simulink model "Hexa_ASMC"  (R2023a)
settings: Solver=ode4  StartTime=0.0  StopTime=tf  FixedStep=0.01  RelTol=1e-3
values from neighbouring files (symbols this model uses):
  ArmConstants = struct('l1_dim', l1_dim,                        'l2_dim', l2_dim,                        'Hexa_to_joint_L', L,                        'Mass1', ml1,                        'Mass2', ml2,                        'Inertia1', Hl1,                        'Inertia2', Hl2,                        'MC1', c1,                        'MC2', c2,                        'Servos', Servos)    [init_model.m]
  HexaConstants = struct('Mass', mb,                         'Inertia', J ,                         'invallo', invallo,                         'kT', kT)    [init_model.m]
settings Model: Creator=Jorge  LastModifiedBy=danie
settings DataIOCC: ReturnWorkspaceOutputs=off
settings OptimizationCC: ReuseModelBlockBuffer=off
settings DebuggingCC: UnconnectedInputMsg=warning  UnconnectedOutputMsg=warning  UnconnectedLineMsg=warning
settings ModelReferenceCC: EnableRefExpFcnMdlSchedulingChecks=on
settings RTWCC: DLArmComputeVersion=19.05
settings DiagnosticsConfigSet: SimMechanicsRigidlyBoundBlock=warning
settings ExplorerConfigSet: InternalSimMechanicsExplorerSettings="<ExplorerConfiguration><canonicalview>default</canonicalview><AnimationSetting><BasePlaybackSpeed>1.0</BasePlaybackSpeed><PlaybackSpeedFactor>4.0</PlaybackSpeedFactor></AnimationSetting><TilePanel><TileInfo><Tiles Columns=\"1\" Count=\"1\" Rows=\"1\"><Column Weight=\"1\"/><Row Weight=\"1\"/><Tile Height=\"1\" Width=\"1\" X=\"0\" Y=\"0\"/></Tiles></TileInfo><SceneInfo><SceneViewer><BGColor><R>0.60000002384185791</R><G>0.60000002384185791</G><B>0.60000002384185791</B></BGColor><Camera><DoPerspective>off</DoPerspective><Position><X>-3.90727997960079421</X><Y>2.05428323506579513</Y><Z>1.78515478561793706</Z></Position><Center><X>0.0641025917185230748</X><Y>-0.340203768406677431</Y><Z>0.439985738763349676</Z></Center><Up><X>0.2129099347365212</X><Y>-0.185763056293179685</Y><Z>0.959250460832366536</Z></Up><ViewLimDist>1</ViewLimDist><YLim>1.44101175579229102</YLim><XLim>2.86953370221693493</XLim></Camera></SceneViewer></SceneInfo></TilePanel><MechEditorPanel><Cameras/><GfxPanelCameraMap/><VideoCreator><PlaybackSpeedRatio>4.0</PlaybackSpeedRatio><FrameRate>30</FrameRate><VideoFormat>MPEG-4</VideoFormat><FrameSize>[1920 1080]</FrameSize></VideoCreator></MechEditorPanel></ExplorerConfiguration>"

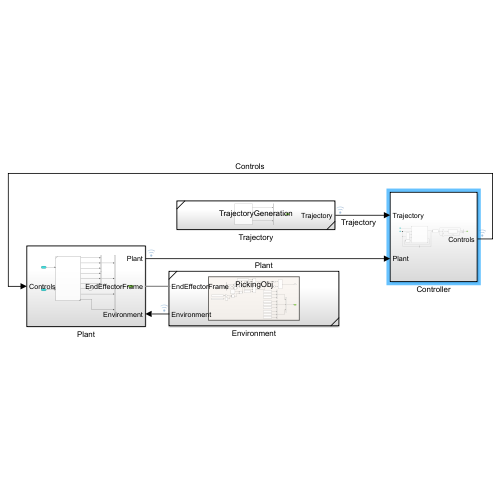
[thumbnail: Simulink's stored preview of the top-level diagram]
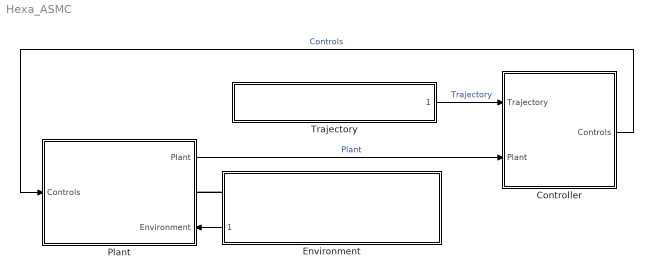
== system Hexa_ASMC ==
  Controller : Subsystem
  Environment : Subsystem  ReferencedSubsystem=PickingObj
      settings: PortSchema="{\"entries\":[{\"content\":{\"sides\":[{\"content\":{\"connectorIds\":[\"LConn1\",\"Out1\"]},\"type\":\"ConnectorPlacement.EquallySpacedRectSide\",\"uuid\":\"5c08cfce-bb37-47ad-9aee-09cd3d0a9d82\"},{\"content\":{\"side\":\"RIGHT\"},\"type\":\"ConnectorPlacement.EquallySpacedRectSide\",\"uuid\":\"54293c39-26a9-438b-b1f6-8d0b93a0680a\"},{\"content\":{\"side\":\"TOP\"},\"type\":\"ConnectorPlacement.EquallySpacedRectSide\",\"uuid\":\"14552c0b-480b-4ef8-a964-bf21c28e2914\"}]},\"type\":\"ConnectorPlacement.EquallySpacedConnector\",\"uuid\":\"e6e3027e-622b-4c2e-b3cf-73a625fb57e1\"}],\"packageUris\":[\"http://schema.mathworks.com/mf0/Connector/R2020b\"],\"version\":\"1.0\"}"
  Plant : Subsystem
      settings: PortSchema="{\"entries\":[{\"content\":{\"sides\":[{\"content\":{\"connectorIds\":[\"In1\"]},\"type\":\"ConnectorPlacement.EquallySpacedRectSide\",\"uuid\":\"11bcd53b-55b2-4d69-a1dd-85bd17ae1b26\"},{\"content\":{\"connectorIds\":[\"Out1\",\"RConn1\",\"In2\"],\"side\":\"RIGHT\"},\"type\":\"ConnectorPlacement.EquallySpacedRectSide\",\"uuid\":\"8deb2c99-cdf2-4c07-9bda-82202a10127f\"},{\"content\":{\"side\":\"TOP\"},\"type\":\"ConnectorPlacement.EquallySpacedRectSide\",\"uuid\":\"e1cee1e1-f12a-4bbb-be1b-b1297a2f8e40\"}]},\"type\":\"ConnectorPlacement.EquallySpacedConnector\",\"uuid\":\"11daab03-d64c-4920-b3ce-5e6ee12e0c1c\"}],\"packageUris\":[\"http://schema.mathworks.com/mf0/Connector/R2020b\"],\"version\":\"1.0\"}"
  Trajectory : Subsystem  ReferencedSubsystem=TrajectoryGeneration
  wires:
  Trajectory/1 -> Controller/1(Trajectory)  "Trajectory"
  Controller/1(Controls) -> Plant/1(Controls)  "Controls"
  Plant/1(Plant) -> Controller/2(Plant)  "Plant"
  Environment/1 -> Plant/2(Environment)
  connections:
  Environment/LConn1 -- Plant/RConn1

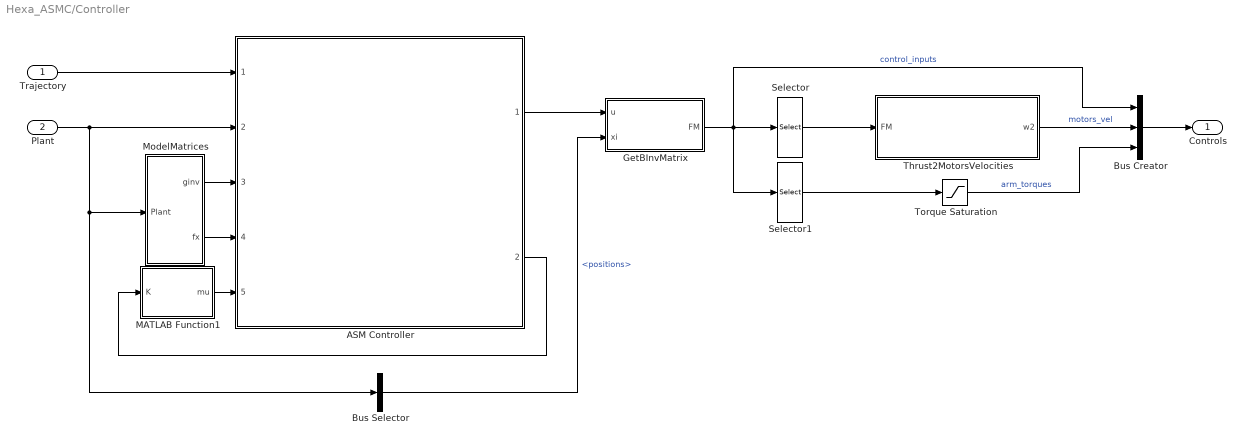
== system Hexa_ASMC/Controller ==
  Trajectory : Inport
  Plant : Inport  Port=2  OutDataTypeStr=Bus: PlantBusDef
  ASM Controller : Subsystem  ReferencedSubsystem=ASMController
  Bus Creator : BusCreator  Inputs=3
  Bus Selector : BusSelector  OutputSignals=positions
  GetBInvMatrix : MATLAB Function  TreatAsAtomicUnit=on
  MATLAB Function1 : MATLAB Function  TreatAsAtomicUnit=on
  ModelMatrices : Subsystem
  Selector : Selector  InputPortWidth=8  IndexOptions=Index vector (dialog)  Indices=1:6  OutputSizes=1
  Selector1 : Selector  InputPortWidth=8  IndexOptions=Index vector (dialog)  Indices=7:8  OutputSizes=1
  Thrust2MotorsVelocities : Subsystem
  Torque Saturation : Saturate  UpperLimit=ArmConstants.Servos.T1max  LowerLimit=-ArmConstants.Servos.T1max
  Controls : Outport  OutDataTypeStr=Bus: ControlsBusDef
  wires:
  Selector/1 -> Thrust2MotorsVelocities/1(FM)
  Selector1/1 -> Torque Saturation/1
  GetBInvMatrix/1(FM) -> Bus Creator/1, Selector1/1, Selector/1  "control_inputs"
  Plant/1 -> Bus Selector/1, ModelMatrices/1(Plant), ASM Controller/2
  Bus Selector/1 -> GetBInvMatrix/2(xi)  "<positions>"
  Torque Saturation/1 -> Bus Creator/3  "arm_torques"
  Thrust2MotorsVelocities/1(w2) -> Bus Creator/2  "motors_vel"
  Bus Creator/1 -> Controls/1
  ASM Controller/2 -> MATLAB Function1/1(K)
  Trajectory/1 -> ASM Controller/1
  ASM Controller/1 -> GetBInvMatrix/1(u)
  ModelMatrices/1(ginv) -> ASM Controller/3
  ModelMatrices/2(fx) -> ASM Controller/4
  MATLAB Function1/1(mu) -> ASM Controller/5

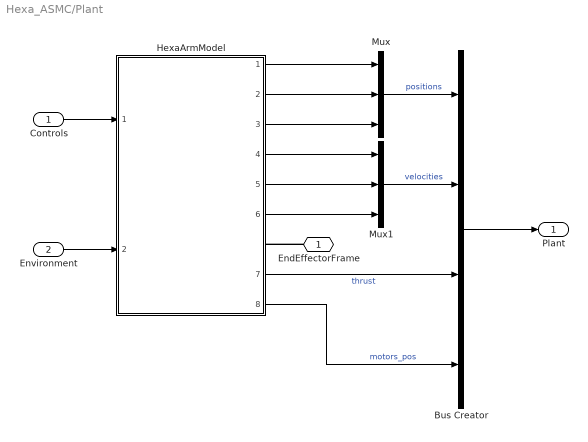
== system Hexa_ASMC/Plant ==
  Controls : Inport  OutDataTypeStr=Bus: ControlsBusDef
  Environment : Inport  Port=2  OutDataTypeStr=Bus: EnvironmentBusDef
  Bus Creator : BusCreator  Inputs=4
  HexaArmModel : Subsystem  ReferencedSubsystem=HexaArmModel
      settings: PortSchema="{\"entries\":[{\"content\":{\"sides\":[{\"content\":{\"connectorIds\":[\"In1\",\"In2\"]},\"type\":\"ConnectorPlacement.EquallySpacedRectSide\",\"uuid\":\"2dc8ce6a-8c2d-483c-b9eb-4519b8adf1d0\"},{\"content\":{\"connectorIds\":[\"Out1\",\"Out2\",\"Out3\",\"Out4\",\"Out5\",\"Out6\",\"LConn1\",\"Out7\",\"Out8\"],\"side\":\"RIGHT\"},\"type\":\"ConnectorPlacement.EquallySpacedRectSide\",\"uuid\":\"8919d7d9-a4a6-435e-91a0-6baaf43bb5dd\"},{\"content\":{\"side\":\"TOP\"},\"type\":\"ConnectorPlacement.EquallySpacedRectSide\",\"uuid\":\"fa3a5bef-28de-4da0-87cc-ec475f477ce4\"},{\"content\":{\"side\":\"BOTTOM\"},\"type\":\"ConnectorPlacement.EquallySpacedRectSide\",\"uuid\":\"150f6a32-8ea9-4dd2-b567-bcfc66bb4dd6\"}]},\"type\":\"ConnectorPlacement.EquallySpacedConnector\",\"uuid\":\"31c51f19-2717-4f79-8154-231ed584b48f\"}],\"packageUris\":[\"http://schema.mathworks.com/mf0/Connector/R2020b\"],\"version\":\"1.0\"}"
  Mux : Mux  Inputs=3
  Mux1 : Mux  Inputs=3
  EndEffectorFrame : PMIOPort  Side=Right
  Plant : Outport  OutDataTypeStr=Bus: PlantBusDef
  wires:
  Bus Creator/1 -> Plant/1
  Controls/1 -> HexaArmModel/1
  HexaArmModel/1 -> Mux/1
  HexaArmModel/2 -> Mux/2
  HexaArmModel/3 -> Mux/3
  HexaArmModel/4 -> Mux1/1
  HexaArmModel/5 -> Mux1/2
  HexaArmModel/6 -> Mux1/3
  Mux/1 -> Bus Creator/1  "positions"
  Mux1/1 -> Bus Creator/2  "velocities"
  HexaArmModel/7 -> Bus Creator/3  "thrust"
  Environment/1 -> HexaArmModel/2
  HexaArmModel/8 -> Bus Creator/4  "motors_pos"
  connections:
  EndEffectorFrame/RConn1 -- HexaArmModel/LConn1

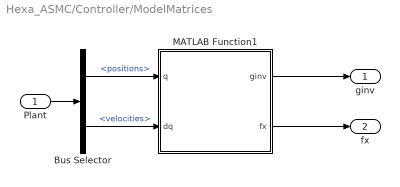
== system Hexa_ASMC/Controller/ModelMatrices ==
  Plant : Inport
  Bus Selector : BusSelector  OutputSignals=positions,velocities
  MATLAB Function1 : MATLAB Function  TreatAsAtomicUnit=on
  ginv : Outport
  fx : Outport  Port=2
  wires:
  Bus Selector/1 -> MATLAB Function1/1(q)  "<positions>"
  Bus Selector/2 -> MATLAB Function1/2(dq)  "<velocities>"
  Plant/1 -> Bus Selector/1
  MATLAB Function1/1(ginv) -> ginv/1
  MATLAB Function1/2(fx) -> fx/1

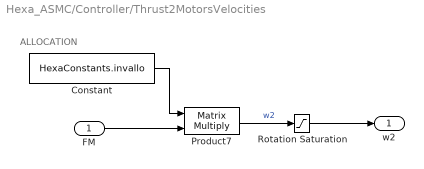
== system Hexa_ASMC/Controller/Thrust2MotorsVelocities ==
  note: ALLOCATION
  FM : Inport
  Constant : Constant  Value=HexaConstants.invallo
  Product7 : Product  Multiplication=Matrix(*)
  Rotation Saturation : Saturate  UpperLimit=8.77e+05  LowerLimit=0
  w2 : Outport
  wires:
  FM/1 -> Product7/2
  Constant/1 -> Product7/1
  Product7/1 -> Rotation Saturation/1  "w2"
  Rotation Saturation/1 -> w2/1

== matlab function Hexa_ASMC/Controller/GetBInvMatrix ==
  data: u input; xi input; FM output
function FM = GetBInvMatrix(u,xi)

% phi = xi(4);
% th  = xi(5);
% psi = xi(6);
% 
% BM1=[cos(phi)*cos(th),-cos(phi)*sin(psi)+cos(psi)*sin(phi)*sin(th), ...
%     sin(phi)*sin(psi)+cos(phi)*cos(psi)*sin(th),0,0,0;...
%     cos(th)*sin(psi), cos(phi)*cos(psi)+sin(phi)*sin(psi)*sin(th),...
%     -cos(psi)*sin(phi)+cos(phi)*sin(psi)*sin(phi),0,0,0;...
%     -sin(th),cos(th)*sin(psi),cos(phi)*cos(th),0,0,0;...
%     0,0,0,1,sin(phi)*tan(th),cos(phi)*tan(th);...
%     0,0,0,0,cos(phi),-sin(phi);0,0,0,0,sec(th)*sin(phi),cos(phi)*sec(th)];

BM1 = BMatrix(xi);

BM = blkdiag(BM1, eye(2,2));

FM = BM\u;

end

== matlab function Hexa_ASMC/Controller/MATLAB Function1 ==
  data: K input; mu output; ASMC parameter
function mu = mu_func(K, ASMC)

muw = 4 * 0.01 * ones(size(K));
mu =  muw .* K;

idx = mu >= ASMC.mu;

mu(idx) = ASMC.mu(idx);

end

== matlab function Hexa_ASMC/Controller/ModelMatrices/MATLAB Function1 ==
  data: q input; dq input; HexaConstants parameter; ginv output; fx output; ArmConstants parameter
function [ginv, fx] = Get_DCG_Hexa(q, dq, HexaConstants, ArmConstants)

DM = DMatrix(q, HexaConstants, ArmConstants);
CM = CMatrix(q, dq, HexaConstants, ArmConstants);
Gv = GVector(q, HexaConstants, ArmConstants);

ginv = DM;

fx = DM\( -CM*dq - Gv );

end
